simulink model "ComfortMdLStEnCtrl"  (R2018b)
settings: Solver=FixedStepDiscrete  StartTime=0.0  StopTime=10.0  FixedStep=0.01  RelTol=1e-3
undefined symbols (not defined in the file or in its folder): data, KeSMSw4SSecRwLtStLgrstOtwdInwdClosePos1_Val, KeSMSw4SSecRwLtStLgrstUpwdDnwdClosePos1_Val, KeSMSw4SSecRwLtStLgrstUpwdDnwdClosePos2_Val, KeSMSw4SSecRwLtStLgrstUpwdDnwdOpenPos1_Val, SecRwLtStBkRclnEn_Clear, SecRwLtStBkRclnEn_Set, SecRwLtStLgrstInwdOtwdEn_Clear, SecRwLtStLgrstInwdOtwdEn_Set, SecRwLtStLgrstUpwdDnwdEn_Clear, SecRwLtStLgrstUpwdDnwdEn_Set, ZeroLEn_Clear, ZeroLEn_Set
libraries: simulink x1
settings Model: Creator=sn2xws  LastModifiedBy=sn55gm
settings Model: ModifiedHistory=|
  | 2024.6.19 V1.1.0 模式流程V1.6
  | 2024.8.8 V3.0.0 ALL DONE判断条件变更
settings DataIOCC: SaveFormat=StructureWithTime
settings OptimizationCC: DefaultParameterBehavior=Inlined  EnhancedBackFolding=on  PassReuseOutputArgsAs=Individual arguments  ZeroExternalMemoryAtStartup=off  ZeroInternalMemoryAtStartup=off  OptimizeBlockOrder=speed  DifferentSizesBufferReuse=on  OptimizationCustomize=off
settings DebuggingCC: ParameterTunabilityLossMsg=error
settings SFSimCC: MATLABDynamicMemAlloc=off
settings RTWCC: SystemTargetFile=autosar.tlc  GenCodeOnly=on  TemplateMakefile=ert_default_tmf  Description=AUTOSAR  GenerateReport=on  IncludeHyperlinkInReport=on  LaunchReport=on  GenerateTraceInfo=on  GenerateTraceReport=on  GenerateTraceReportSl=on  GenerateTraceReportSf=on  GenerateTraceReportEml=on
settings CodeAppCC: ForceParamTrailComments=on  IgnoreCustomStorageClasses=off  OperatorAnnotations=on  SimulinkDataObjDesc=on  SFDataObjDesc=on  InsertBlockDesc=on
settings STFCustomTargetCC: TargetLangStandard=C99 (ISO)  MultiwordLength=256  ParMdlRefBuildCompliant=on  CompOptLevelCompliant=on  IncludeMdlTerminateFcn=off  CombineOutputUpdateFcns=on  SuppressErrorStatus=on  ERTCustomFileBanners=on  SupportNonFinite=off  SupportComplex=off  SupportContinuousTime=off  SupportNonInlinedSFcns=off  RemoveResetFunc=on  MATLABClassNameForMDSCustomization=Simulink.SoftwareTarget.ERTCustomization  AutosarCompliant=on  UseToolchainInfoCompliant=on  LookupTableObjectStructAxisOrder=2,1,3,4,...  LUTObjectStructOrderEvenSpacing=Size,Table,Breakpoints  SystemTargetFile=autosar.tlc
settings ERTTargetCC: TargetLangStandard=C99 (ISO)  ConcurrentExecutionCompliant=off  IncludeMdlTerminateFcn=off  SuppressErrorStatus=on  SupportNonFinite=off  SupportComplex=off  ModelStepFunctionPrototypeControlCompliant=off  CPPClassGenCompliant=off  AutosarCompliant=on  LookupTableObjectStructAxisOrder=2,1,3,4,...  LUTObjectStructOrderEvenSpacing=Size,Table,Breakpoints  InlinedParameterPlacement=NonHierarchical  ERTCustomFileTemplate=example_file_process.tlc  ERTFilePackagingFormat=Compact

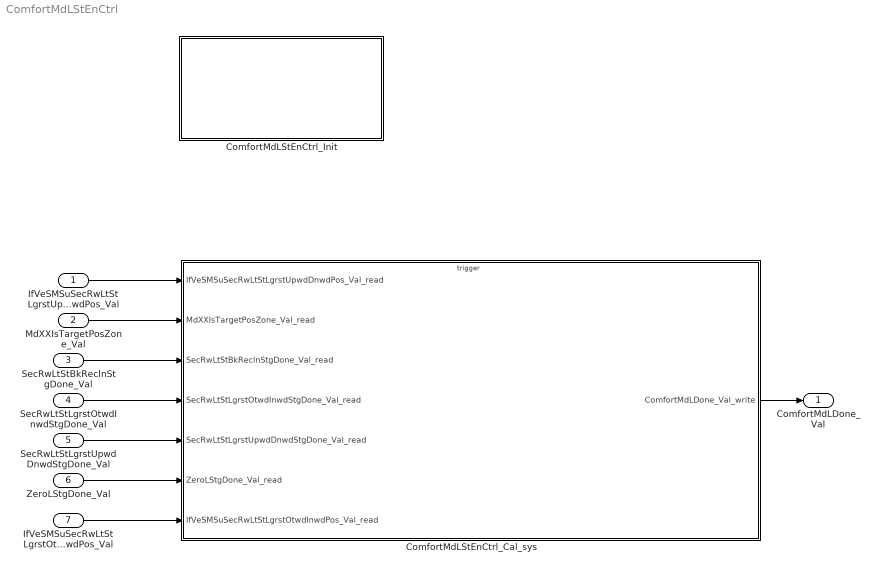
== system ComfortMdLStEnCtrl ==
  IfVeSMSuSecRwLtStLgrstUpwdDnwdPos_Val : Inport  OutDataTypeStr=uint16  PortDimensions=1
  MdXXIsTargetPosZone_Val : Inport  Port=2  OutDataTypeStr=uint32  PortDimensions=1
  SecRwLtStBkReclnStgDone_Val : Inport  Port=3  OutDataTypeStr=boolean  PortDimensions=1
  SecRwLtStLgrstOtwdInwdStgDone_Val : Inport  Port=4  OutDataTypeStr=boolean  PortDimensions=1
  SecRwLtStLgrstUpwdDnwdStgDone_Val : Inport  Port=5  OutDataTypeStr=boolean  PortDimensions=1
  ZeroLStgDone_Val : Inport  Port=6  OutDataTypeStr=boolean  PortDimensions=1
  IfVeSMSuSecRwLtStLgrstOtwdInwdPos_Val : Inport  Port=7  OutDataTypeStr=uint16  PortDimensions=1
  ComfortMdLStEnCtrl_Cal_sys : Subsystem
  ComfortMdLStEnCtrl_Init : Subsystem
  ComfortMdLDone_Val : Outport  OutDataTypeStr=uint8  PortDimensions=1
  wires:
  IfVeSMSuSecRwLtStLgrstUpwdDnwdPos_Val/1 -> ComfortMdLStEnCtrl_Cal_sys/1(IfVeSMSuSecRwLtStLgrstUpwdDnwdPos_Val_read)
  MdXXIsTargetPosZone_Val/1 -> ComfortMdLStEnCtrl_Cal_sys/2(MdXXIsTargetPosZone_Val_read)
  SecRwLtStBkReclnStgDone_Val/1 -> ComfortMdLStEnCtrl_Cal_sys/3(SecRwLtStBkReclnStgDone_Val_read)
  SecRwLtStLgrstOtwdInwdStgDone_Val/1 -> ComfortMdLStEnCtrl_Cal_sys/4(SecRwLtStLgrstOtwdInwdStgDone_Val_read)
  SecRwLtStLgrstUpwdDnwdStgDone_Val/1 -> ComfortMdLStEnCtrl_Cal_sys/5(SecRwLtStLgrstUpwdDnwdStgDone_Val_read)
  ZeroLStgDone_Val/1 -> ComfortMdLStEnCtrl_Cal_sys/6(ZeroLStgDone_Val_read)
  ComfortMdLStEnCtrl_Cal_sys/1(ComfortMdLDone_Val_write) -> ComfortMdLDone_Val/1
  IfVeSMSuSecRwLtStLgrstOtwdInwdPos_Val/1 -> ComfortMdLStEnCtrl_Cal_sys/7(IfVeSMSuSecRwLtStLgrstOtwdInwdPos_Val_read)

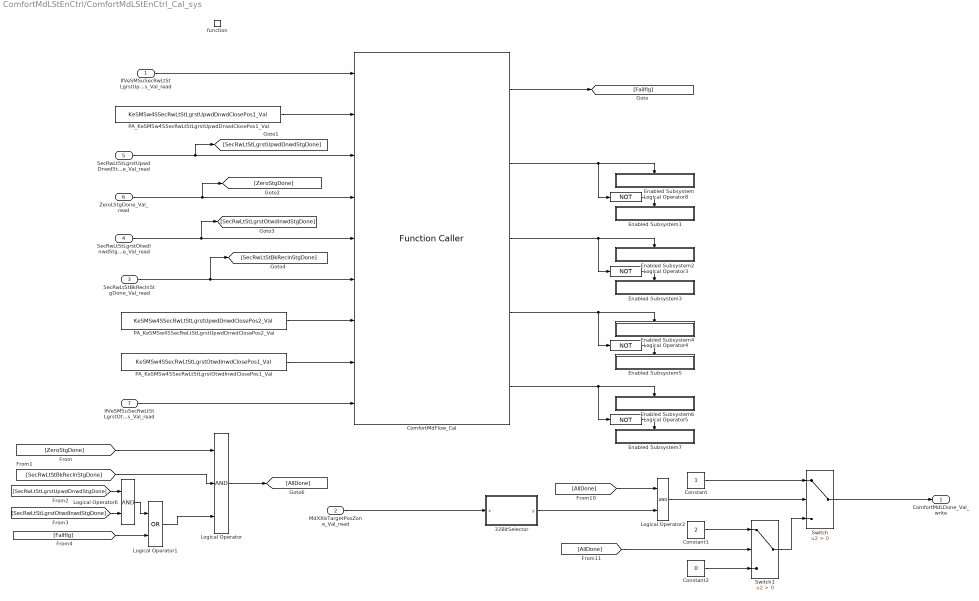
== system ComfortMdLStEnCtrl/ComfortMdLStEnCtrl_Cal_sys ==
  IfVeSMSuSecRwLtStLgrstUpwdDnwdPos_Val_read : Inport
  MdXXIsTargetPosZone_Val_read : Inport  Port=2
  SecRwLtStBkReclnStgDone_Val_read : Inport  Port=3
  SecRwLtStLgrstOtwdInwdStgDone_Val_read : Inport  Port=4
  SecRwLtStLgrstUpwdDnwdStgDone_Val_read : Inport  Port=5
  ZeroLStgDone_Val_read : Inport  Port=6
  IfVeSMSuSecRwLtStLgrstOtwdInwdPos_Val_read : Inport  Port=7
  function : TriggerPort  TriggerType=function-call  IsSimulinkFunction=on  FunctionName=ComfortMdLStEnCtrl_Cal  VariantControl=(inherit)
  32BitSelector : Subsystem  mask(32 Bit Selector){BitNum=10}
      mask prompts: BitNum "Select Bit Number"
      mask help: Allows selection of a particular bit (0-31) out of a packed word up to 32 bits long. Output will be true if the bit number selected via the mask parameter is equal to one.
      mask TypeOptions BitNum: 0 | 1 | 2 | 3 | 4 | 5 | 6 | 7 | 8 | 9 | 10 | 11 | 12 | 13 | 14 | 15 | 16 | 17 | 18 | 19 | 20 | 21 | 22 | 23 | 24 | 25 | 26 | 27 | 28 | 29 | 30 | 31
      mask Display:
      | text(0.5, 0.8,'BIT','horizontalAlignment','center')
      | text(0.5, 0.5,'SELECTOR','horizontalAlignment','center')
      | text(0.5, 0.2,['-- Bit ',char(get_param(gcb,'BitNum')),' --'],'horizontalAlignment','center')
  ComfortMdFlow_Cal : FunctionCaller  FunctionPrototype=[Failflg,LgrstInwdOtwdEn,LgrstUpwdDnwdEn,ZeroEn,BkReclnEn] = ComfortMdFlow_Cal(LgrstUpwdDnwdPos,LgrstUpwdDnwdClosePos1,LgrstUpwdStgDone,ZeroStgDone,LgrstInwdStgDone,BkReclnStgDone,LgrstUpwdDnwdClosePos2,LgrstInwdOtwdClosePos1,LgrstInwdOtwdPos)  InputArgumentSpecifications=uint16(1), uint16(1), boolean(true), boolean(true), boolean(true), boolean(true), uint16(1), uint16(1), uint16(1)  OutputArgumentSpecifications=boolean(true), boolean(true), boolean(true), boolean(true), boolean(true)
  Constant : Constant  OutDataTypeStr=uint8
  Constant1 : Constant  Value=2  OutDataTypeStr=uint8
  Constant2 : Constant  Value=0  OutDataTypeStr=uint8
  Enabled Subsystem : Subsystem  TreatAsAtomicUnit=on
  Enabled Subsystem1 : Subsystem  TreatAsAtomicUnit=on
  Enabled Subsystem2 : Subsystem  TreatAsAtomicUnit=on
  Enabled Subsystem3 : Subsystem  TreatAsAtomicUnit=on
  Enabled Subsystem4 : Subsystem  TreatAsAtomicUnit=on
  Enabled Subsystem5 : Subsystem  TreatAsAtomicUnit=on
  Enabled Subsystem6 : Subsystem  TreatAsAtomicUnit=on
  Enabled Subsystem7 : Subsystem  TreatAsAtomicUnit=on
  Logical Operator : Logic  Inputs=3  AllPortsSameDT=off  OutDataTypeStr=boolean
  Logical Operator1 : Logic  Operator=OR  AllPortsSameDT=off  OutDataTypeStr=boolean
  Logical Operator2 : Logic  AllPortsSameDT=off  OutDataTypeStr=boolean
  Logical Operator{3..5,8} (4 alike) : Logic  Operator=NOT  AllPortsSameDT=off  OutDataTypeStr=boolean
  Logical Operator6 : Logic  AllPortsSameDT=off  OutDataTypeStr=boolean
  PA_KeSMSw4SSecRwLtStLgrstOtwdInwdClosePos1_Val : Constant  Value=KeSMSw4SSecRwLtStLgrstOtwdInwdClosePos1_Val
  PA_KeSMSw4SSecRwLtStLgrstUpwdDnwdClosePos1_Val : Constant  Value=KeSMSw4SSecRwLtStLgrstUpwdDnwdClosePos1_Val
  PA_KeSMSw4SSecRwLtStLgrstUpwdDnwdClosePos2_Val : Constant  Value=KeSMSw4SSecRwLtStLgrstUpwdDnwdClosePos2_Val
  Switch : Switch  Criteria=u2 > Threshold
  Switch1 : Switch  Criteria=u2 > Threshold
  ComfortMdLDone_Val_write : Outport
      settings: EnsureOutportIsVirtual=on
  wires:
  IfVeSMSuSecRwLtStLgrstUpwdDnwdPos_Val_read/1 -> ComfortMdFlow_Cal/1
  SecRwLtStLgrstUpwdDnwdStgDone_Val_read/1 -> [SecRwLtStLgrstUpwdDnwdStgDone], ComfortMdFlow_Cal/3
  ZeroLStgDone_Val_read/1 -> [ZeroStgDone], ComfortMdFlow_Cal/4
  SecRwLtStLgrstOtwdInwdStgDone_Val_read/1 -> [SecRwLtStLgrstOtwdInwdStgDone], ComfortMdFlow_Cal/5
  SecRwLtStBkReclnStgDone_Val_read/1 -> [SecRwLtStBkReclnStgDone], ComfortMdFlow_Cal/6
  ComfortMdFlow_Cal/1 -> [Failflg]
  [ZeroStgDone] -> Logical Operator/1
  [SecRwLtStBkReclnStgDone] -> Logical Operator/2
  Logical Operator1/1 -> Logical Operator/3
  ComfortMdFlow_Cal/2 -> Logical Operator8/1, Enabled Subsystem/Enable
  Logical Operator8/1 -> Enabled Subsystem1/Enable
  Logical Operator/1 -> [AllDone]
  Switch/1 -> ComfortMdLDone_Val_write/1
  [AllDone] -> Logical Operator2/1
  Switch1/1 -> Switch/3
  MdXXIsTargetPosZone_Val_read/1 -> 32BitSelector/1(x)
  Constant1/1 -> Switch1/1
  Constant2/1 -> Switch1/3
  Logical Operator2/1 -> Switch/2
  [AllDone] -> Switch1/2
  32BitSelector/1(y) -> Logical Operator2/2
  Constant/1 -> Switch/1
  Logical Operator3/1 -> Enabled Subsystem3/Enable
  ComfortMdFlow_Cal/3 -> Logical Operator3/1, Enabled Subsystem2/Enable
  ComfortMdFlow_Cal/4 -> Enabled Subsystem4/Enable, Logical Operator4/1
  Logical Operator4/1 -> Enabled Subsystem5/Enable
  Logical Operator5/1 -> Enabled Subsystem7/Enable
  ComfortMdFlow_Cal/5 -> Logical Operator5/1, Enabled Subsystem6/Enable
  [Failflg] -> Logical Operator1/2
  PA_KeSMSw4SSecRwLtStLgrstUpwdDnwdClosePos2_Val/1 -> ComfortMdFlow_Cal/7
  IfVeSMSuSecRwLtStLgrstOtwdInwdPos_Val_read/1 -> ComfortMdFlow_Cal/9
  [SecRwLtStLgrstOtwdInwdStgDone] -> Logical Operator6/2
  [SecRwLtStLgrstUpwdDnwdStgDone] -> Logical Operator6/1
  Logical Operator6/1 -> Logical Operator1/1
  PA_KeSMSw4SSecRwLtStLgrstOtwdInwdClosePos1_Val/1 -> ComfortMdFlow_Cal/8
  PA_KeSMSw4SSecRwLtStLgrstUpwdDnwdClosePos1_Val/1 -> ComfortMdFlow_Cal/2

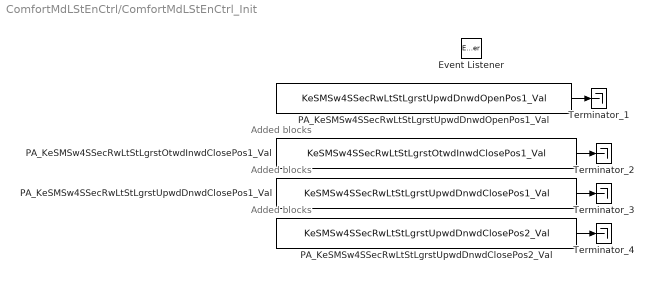
== system ComfortMdLStEnCtrl/ComfortMdLStEnCtrl_Init ==
  note: Added blocks
  note: Added blocks
  note: Added blocks
  Event Listener : EventListener  EventName=reset
  PA_KeSMSw4SSecRwLtStLgrstOtwdInwdClosePos1_Val : Constant  Value=KeSMSw4SSecRwLtStLgrstOtwdInwdClosePos1_Val
  PA_KeSMSw4SSecRwLtStLgrstUpwdDnwdClosePos1_Val : Constant  Value=KeSMSw4SSecRwLtStLgrstUpwdDnwdClosePos1_Val
  PA_KeSMSw4SSecRwLtStLgrstUpwdDnwdClosePos2_Val : Constant  Value=KeSMSw4SSecRwLtStLgrstUpwdDnwdClosePos2_Val
  PA_KeSMSw4SSecRwLtStLgrstUpwdDnwdOpenPos1_Val : Constant  Value=KeSMSw4SSecRwLtStLgrstUpwdDnwdOpenPos1_Val
  Terminator_{1..4} (4 alike) : Terminator
  wires:
  PA_KeSMSw4SSecRwLtStLgrstUpwdDnwdOpenPos1_Val/1 -> Terminator_1/1
  PA_KeSMSw4SSecRwLtStLgrstOtwdInwdClosePos1_Val/1 -> Terminator_2/1
  PA_KeSMSw4SSecRwLtStLgrstUpwdDnwdClosePos1_Val/1 -> Terminator_3/1
  PA_KeSMSw4SSecRwLtStLgrstUpwdDnwdClosePos2_Val/1 -> Terminator_4/1

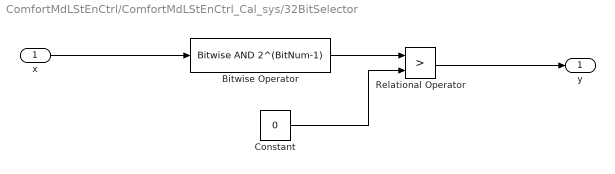
== system ComfortMdLStEnCtrl/ComfortMdLStEnCtrl_Cal_sys/32BitSelector ==
  x : Inport
  Bitwise Operator : simulink/Logic and Bit Operations/Bitwise Operator  logicop=AND  UseBitMask=on  BitMask=2^(BitNum-1)  BitMaskRealWorld=Stored Integer
  Constant : Constant  Value=0  OutDataTypeStr=uint32
  Relational Operator : RelationalOperator  Operator=>  OutDataTypeStr=boolean  RndMeth=Simplest
  y : Outport
  wires:
  Relational Operator/1 -> y/1
  Constant/1 -> Relational Operator/2
  x/1 -> Bitwise Operator/1
  Bitwise Operator/1 -> Relational Operator/1

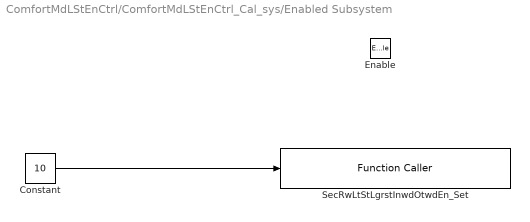
== system ComfortMdLStEnCtrl/ComfortMdLStEnCtrl_Cal_sys/Enabled Subsystem ==
  Enable : EnablePort
  Constant : Constant  Value=10  OutDataTypeStr=uint8
  SecRwLtStLgrstInwdOtwdEn_Set : FunctionCaller  FunctionPrototype=SecRwLtStLgrstInwdOtwdEn_Set(data)  InputArgumentSpecifications=uint8(1)
  wires:
  Constant/1 -> SecRwLtStLgrstInwdOtwdEn_Set/1

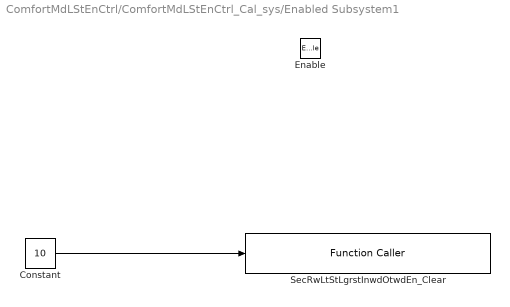
== system ComfortMdLStEnCtrl/ComfortMdLStEnCtrl_Cal_sys/Enabled Subsystem1 ==
  Enable : EnablePort
  Constant : Constant  Value=10  OutDataTypeStr=uint8
  SecRwLtStLgrstInwdOtwdEn_Clear : FunctionCaller  FunctionPrototype=SecRwLtStLgrstInwdOtwdEn_Clear(data)  InputArgumentSpecifications=uint8(1)
  wires:
  Constant/1 -> SecRwLtStLgrstInwdOtwdEn_Clear/1

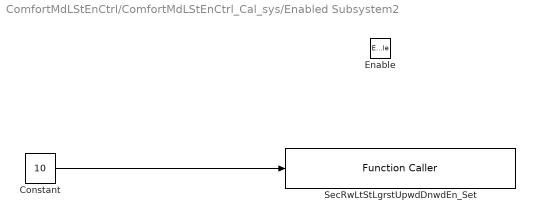
== system ComfortMdLStEnCtrl/ComfortMdLStEnCtrl_Cal_sys/Enabled Subsystem2 ==
  Enable : EnablePort
  Constant : Constant  Value=10  OutDataTypeStr=uint8
  SecRwLtStLgrstUpwdDnwdEn_Set : FunctionCaller  FunctionPrototype=SecRwLtStLgrstUpwdDnwdEn_Set(data)  InputArgumentSpecifications=uint8(1)
  wires:
  Constant/1 -> SecRwLtStLgrstUpwdDnwdEn_Set/1

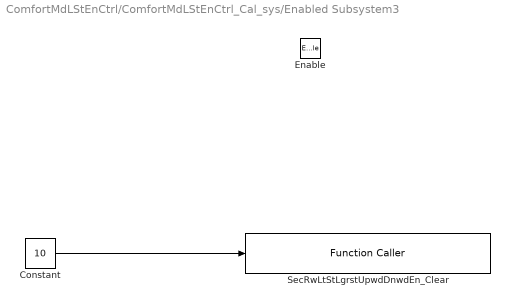
== system ComfortMdLStEnCtrl/ComfortMdLStEnCtrl_Cal_sys/Enabled Subsystem3 ==
  Enable : EnablePort
  Constant : Constant  Value=10  OutDataTypeStr=uint8
  SecRwLtStLgrstUpwdDnwdEn_Clear : FunctionCaller  FunctionPrototype=SecRwLtStLgrstUpwdDnwdEn_Clear(data)  InputArgumentSpecifications=uint8(1)
  wires:
  Constant/1 -> SecRwLtStLgrstUpwdDnwdEn_Clear/1

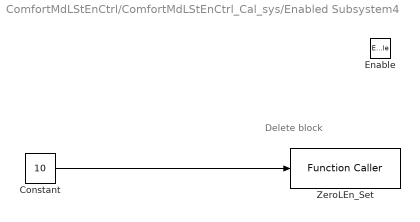
== system ComfortMdLStEnCtrl/ComfortMdLStEnCtrl_Cal_sys/Enabled Subsystem4 ==
  note: Delete block
  Enable : EnablePort
  Constant : Constant  Value=10  OutDataTypeStr=uint8
  ZeroLEn_Set : FunctionCaller  FunctionPrototype=ZeroLEn_Set(data)  InputArgumentSpecifications=uint8(1)
  wires:
  Constant/1 -> ZeroLEn_Set/1

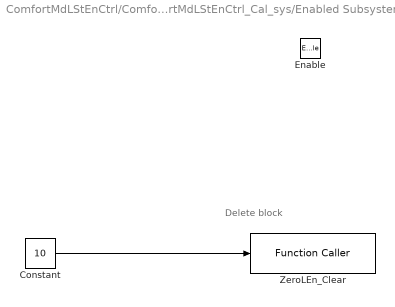
== system ComfortMdLStEnCtrl/ComfortMdLStEnCtrl_Cal_sys/Enabled Subsystem5 ==
  note: Delete block
  Enable : EnablePort
  Constant : Constant  Value=10  OutDataTypeStr=uint8
  ZeroLEn_Clear : FunctionCaller  FunctionPrototype=ZeroLEn_Clear(data)  InputArgumentSpecifications=uint8(1)
  wires:
  Constant/1 -> ZeroLEn_Clear/1

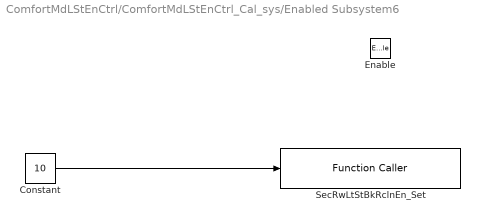
== system ComfortMdLStEnCtrl/ComfortMdLStEnCtrl_Cal_sys/Enabled Subsystem6 ==
  Enable : EnablePort
  Constant : Constant  Value=10  OutDataTypeStr=uint8
  SecRwLtStBkRclnEn_Set : FunctionCaller  FunctionPrototype=SecRwLtStBkRclnEn_Set(data)  InputArgumentSpecifications=uint8(1)
  wires:
  Constant/1 -> SecRwLtStBkRclnEn_Set/1

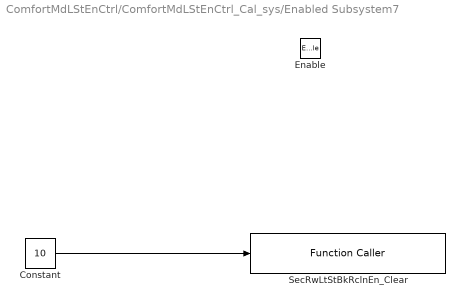
== system ComfortMdLStEnCtrl/ComfortMdLStEnCtrl_Cal_sys/Enabled Subsystem7 ==
  Enable : EnablePort
  Constant : Constant  Value=10  OutDataTypeStr=uint8
  SecRwLtStBkRclnEn_Clear : FunctionCaller  FunctionPrototype=SecRwLtStBkRclnEn_Clear(data)  InputArgumentSpecifications=uint8(1)
  wires:
  Constant/1 -> SecRwLtStBkRclnEn_Clear/1
